simulink model "solution"  (R2017b)
settings: Solver=VariableStepAuto  StartTime=0.0  StopTime=25  FixedStep=0.01  RelTol=1e-3
libraries: simulink x3
settings Model: Creator=ashwin.ramanujam  LastModifiedBy=Vjekoslav

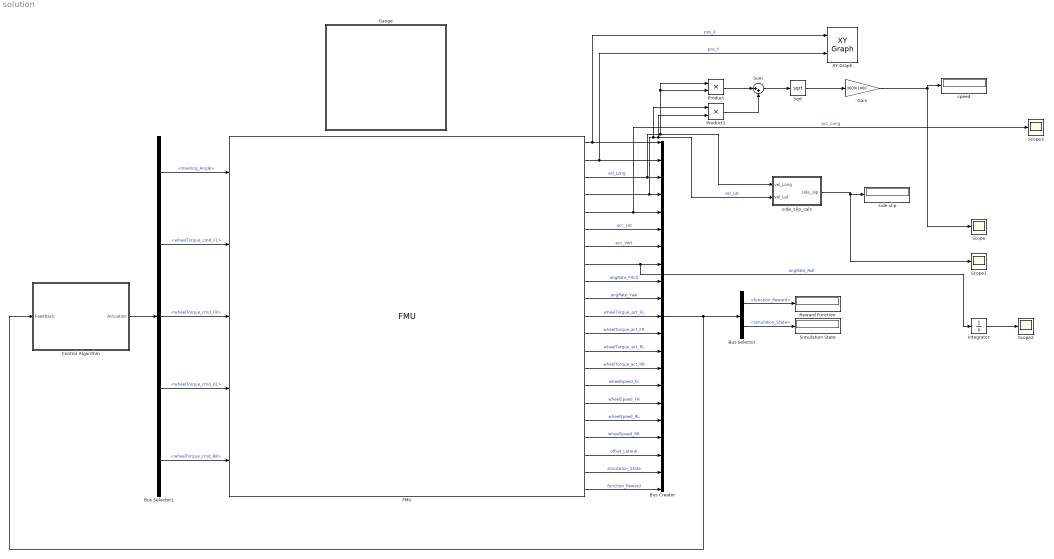
== system solution ==
  Bus Creator : BusCreator  Inputs=21
  Bus Selector : BusSelector  OutputSignals=function_Reward,simulation_State
  Bus Selector1 : BusSelector  OutputSignals=steering_Angle,wheelTorque_cmd_FL,wheelTorque_cmd_FR,wheelTorque_cmd_RL,wheelTorque_cmd_RR
  Control Algorithm : Subsystem
  FMU : FMU  FMUName=MED2018_VehicleModel.fmu  FMUDebugLogging=on  FMUMode=CoSimulation  FMUSampleTime=-1  mask(MED2018.VehicleModel [Co-Simulation, v2.0]){}
      mask Display:
      | if (exist([Simulink.fileGenControl('get','CacheFolder') '\slprj\_fmu\4898b8570ed7ce0a5f76050f8aadaa4c\MED2018_VehicleModel\model.png'],'file'))
      |     image([Simulink.fileGenControl('get','CacheFolder') '\slprj\_fmu\4898b8570ed7ce0a5f76050f8aadaa4c\MED2018_VehicleModel\model.png']);
      |     text(0.03, 0.97, 'MED2018.VehicleModel', 'horizontalAlignment', 'left', 'verticalAlignment', 'top');
      | else
      |     disp('MED2018.VehicleModel');
      | end
      | port_label('output',1,'pos_X');
      | port_label('output',2,'pos_Y');
      | port_label('output',3,'vel_Long');
      | port_label('output',4,'vel_Lat');
      | port_label('output',5,'acc_Long');
      | port_label('output',6,'acc_Lat');
      | port_label('output',7,'acc_Vert');
      | port_label('output',8,'angRate_Roll');
      | port_label('output',9,'angRate_Pitch');
      | port_label('output',10,'angRate_Yaw');
      | port_label('output',11,'wheellTorque_act_FL');
      | port_label('output',12,'wheelTorque_act_FR');
      | port_label('output',13,'wheelTorque_act_RL');
      | port_label('output',14,'wheelTorque_act_RR');
      | port_label('output',15,'wheelSpeed_FL');
      | port_label('output',16,'wheelSpeed_FR');
      | port_label('output',17,'wheelSpeed_RL');
      | port_label('output',18,'wheelSpeed_RR');
      | port_label('output',19,'offset_Lateral');
      | port_label('output',20,'simulation_State');
      | port_label('output',21,'function_Reward');
      | port_label('input',1,'steering_Angle');
      | port_label('input',2,'wheelTorque_cmd_FL');
      | port_label('input',3,'wheelTorque_cmd_FR');
      | port_label('input',4,'wheelTorque_cmd_RL');
      | port_label('input',5,'wheelTorque_cmd_RR');
  Gain : Gain  Gain=3600/1000
  Gauge : Subsystem  DialogController=hmiCreateDDGDialog  IsWebBlock=on  mask(MWDashboardBlock){webBlockId=95ecb222-2df1-432b-9766-14efc8d26a24, webBlockType=circulargauge, ShowInLibBrowser=on, ShowInitialText=on, HMISrcModelName=solution}
      mask prompts: webBlockId "WebBlock Id"; webBlockType "WebBlock Type"; HMISrcModelName "Source Model"
      mask help: SimulinkHMI:dialogs:CircularGaugeDialogDesc
      mask Help: helpview([docroot '/mapfiles/simulink.map'], 'hmi_gauge')
      mask Display:
      | if strcmp(get_param(bdroot(gcb),'BlockDiagramType'), 'library')
      |     image([(matlabroot) '/toolbox/simulink/hmi/icons/CircularGauge.png']);
      | end
  Integrator : Integrator
  Product : Product
  Product1 : Product
  Reward Function : Display
  Scope{,1..3} (4 alike) : Scope
  Simulation State : Display
  Sqrt : Sqrt  SaturateOnIntegerOverflow=on
  Sum : Sum  Inputs=|++
  XY Graph : simulink/Sinks/XY Graph  xmin=-100  xmax=200  ymin=-100  ymax=200  st=-1
  "side slip " : Display
  side_slip_calc : Subsystem
  "speed " : Display
  wires:
  Control Algorithm/1(Actuation) -> Bus Selector1/1
  Bus Selector1/1 -> FMU/1  "<steering_Angle>"
  Bus Selector1/2 -> FMU/2  "<wheelTorque_cmd_FL>"
  Bus Selector1/3 -> FMU/3  "<wheelTorque_cmd_FR>"
  Bus Selector1/4 -> FMU/4  "<wheelTorque_cmd_RL>"
  Bus Selector1/5 -> FMU/5  "<wheelTorque_cmd_RR>"
  FMU/1 -> XY Graph/1, Bus Creator/1  "pos_X"
  FMU/2 -> XY Graph/2, Bus Creator/2  "pos_Y"
  FMU/3 -> side_slip_calc/1(vel_Long), Product/2, Product/1, Bus Creator/3  "vel_Long"
  FMU/4 -> Product1/1, side_slip_calc/2(vel_Lat), Product1/2, Bus Creator/4  "vel_Lat"
  FMU/5 -> Scope3/1, Bus Creator/5  "acc_Long"
  FMU/6 -> Bus Creator/6  "acc_Lat"
  FMU/7 -> Bus Creator/7  "acc_Vert"
  FMU/8 -> Integrator/1, Bus Creator/8  "angRate_Roll"
  FMU/9 -> Bus Creator/9  "angRate_Pitch"
  FMU/10 -> Bus Creator/10  "angRate_Yaw"
  FMU/11 -> Bus Creator/11  "wheelTorque_act_FL"
  FMU/12 -> Bus Creator/12  "wheelTorque_act_FR"
  FMU/13 -> Bus Creator/13  "wheelTorque_act_RL"
  FMU/14 -> Bus Creator/14  "wheelTorque_act_RR"
  FMU/15 -> Bus Creator/15  "wheelSpeed_FL"
  FMU/16 -> Bus Creator/16  "wheelSpeed_FR"
  FMU/17 -> Bus Creator/17  "wheelSpeed_RL"
  FMU/18 -> Bus Creator/18  "wheelSpeed_RR"
  FMU/19 -> Bus Creator/19  "offset_Lateral"
  FMU/20 -> Bus Creator/20  "simulation_State"
  FMU/21 -> Bus Creator/21  "function_Reward"
  Bus Creator/1 -> Bus Selector/1, Control Algorithm/1(Feedback)
  Bus Selector/1 -> Reward Function/1  "<function_Reward>"
  Bus Selector/2 -> Simulation State/1  "<simulation_State>"
  Product1/1 -> Sum/2
  Product/1 -> Sum/1
  Sum/1 -> Sqrt/1
  Sqrt/1 -> Gain/1
  Gain/1 -> "speed "/1, Scope/1
  Integrator/1 -> Scope2/1
  side_slip_calc/1(side_slip) -> Scope1/1, "side slip "/1

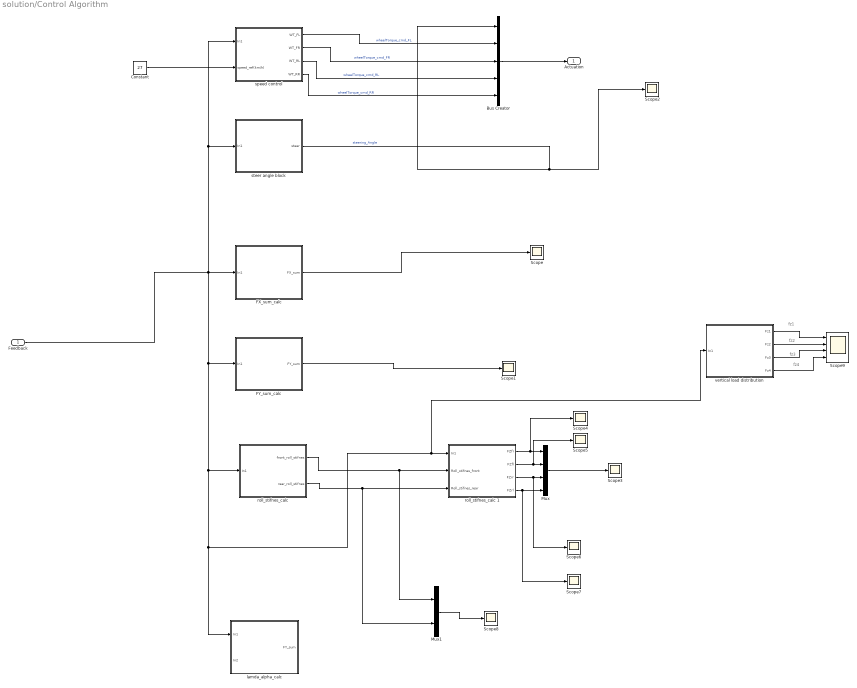
== system solution/Control Algorithm ==
  note: fz3
  note: fz4
  note: fz1
  note: fz2
  Feedback : Inport
  Bus Creator : BusCreator  Inputs=5
  Constant : Constant  Value=27
  FX_sum_calc : Subsystem
  FY_sum_calc : Subsystem
  Mux : Mux
  Mux1 : Mux  Inputs=2
  Scope{,1..8} (9 alike) : Scope
  Scope9 : Scope  NumInputPorts=4
  lamda_alpha_calc : Subsystem
  "roll_stifnes_calc " : Subsystem
  roll_stifnes_calc 1 : Subsystem
  speed control : Subsystem
  "steer angle block " : Subsystem
  vertical load distribution : Subsystem
  Actuation : Outport
  wires:
  speed control/4(WT_RR) -> Bus Creator/5  "wheelTorque_cmd_RR"
  speed control/1("WT_FL ") -> Bus Creator/2  "wheelTorque_cmd_FL"
  speed control/3(WT_RL) -> Bus Creator/4  "wheelTorque_cmd_RL"
  "steer angle block "/1("steer ") -> Scope2/1, Bus Creator/1  "steering_Angle"
  speed control/2(WT_FR) -> Bus Creator/3  "wheelTorque_cmd_FR"
  Bus Creator/1 -> Actuation/1
  FX_sum_calc/1(FX_sum) -> Scope/1
  FY_sum_calc/1(FY_sum) -> Scope1/1
  "roll_stifnes_calc "/1(front_roll_stifnes) -> Mux1/1, roll_stifnes_calc 1/2(Roll_stifnes_front)
  "roll_stifnes_calc "/2(rear_roll_stifnes) -> Mux1/2, roll_stifnes_calc 1/3("Roll_stifnes_rear ")
  Constant/1 -> speed control/2("speed_ref(km/h) ")
  roll_stifnes_calc 1/1(FZfr) -> Scope4/1, Mux/1
  roll_stifnes_calc 1/2(FZfl) -> Scope5/1, Mux/2
  roll_stifnes_calc 1/3(FZrr) -> Scope6/1, Mux/3
  roll_stifnes_calc 1/4(FZrl) -> Scope7/1, Mux/4
  Mux/1 -> Scope3/1
  Mux1/1 -> Scope8/1
  vertical load distribution/3(Fz3) -> Scope9/3
  vertical load distribution/4(Fz4) -> Scope9/4
  vertical load distribution/2(Fz2) -> Scope9/2
  vertical load distribution/1(Fz1) -> Scope9/1
  Feedback/1 -> speed control/1(In1), "steer angle block "/1(In1), FY_sum_calc/1(In1), "roll_stifnes_calc "/1(In1), vertical load distribution/1(In1), roll_stifnes_calc 1/1(In1), lamda_alpha_calc/1(In1), FX_sum_calc/1(In1)

== system solution/Gauge ==

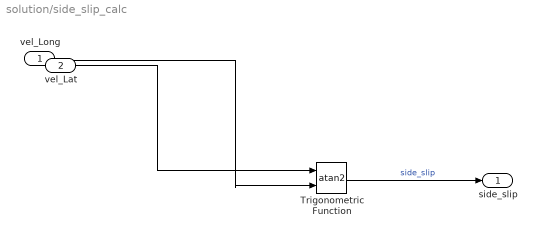
== system solution/side_slip_calc ==
  vel_Long : Inport
  vel_Lat : Inport  Port=2
  Trigonometric Function : Trigonometry  Operator=atan2
  side_slip : Outport
  wires:
  Trigonometric Function/1 -> side_slip/1  "side_slip"
  vel_Lat/1 -> Trigonometric Function/1
  vel_Long/1 -> Trigonometric Function/2

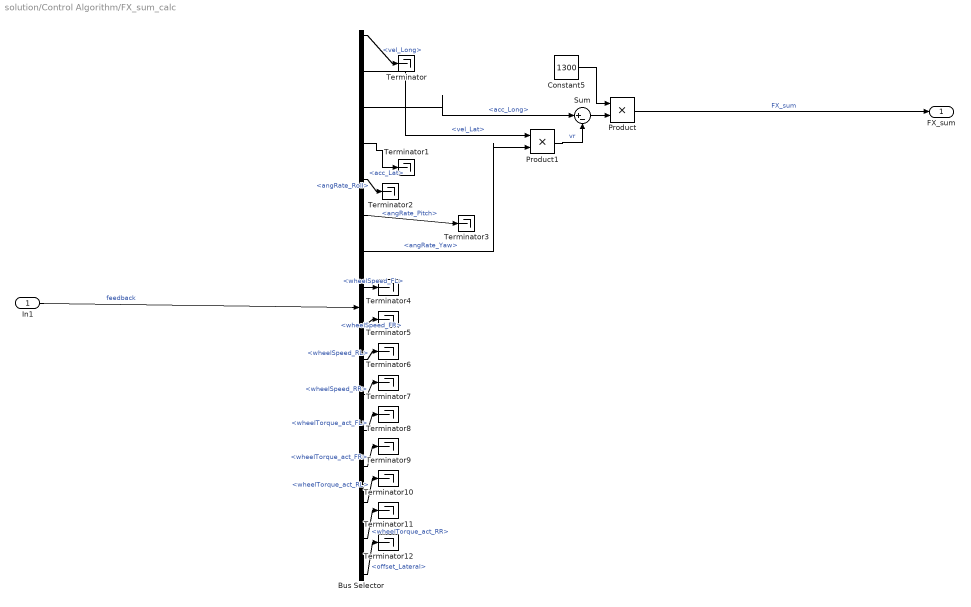
== system solution/Control Algorithm/FX_sum_calc ==
  In1 : Inport
  Bus Selector : BusSelector  OutputSignals=vel_Long,vel_Lat,acc_Long,acc_Lat,angRate_Roll,angRate_Pitch,angRate_Yaw,wheelSpeed_FL,wheelSpeed_FR,wheelSpeed_RL,wheelSpeed_RR,wheelTorque_act_FL,wheelTorque_act_FR,wheelTorque_act_RL,wheelTorque_act_RR,offset_Lateral
  Constant5 : Constant  Value=1300
  Product : Product
  Product1 : Product
  Sum : Sum  Inputs=|+-
  Terminator{,1..12} (13 alike) : Terminator
  FX_sum : Outport
  wires:
  Constant5/1 -> Product/1
  Product1/1 -> Sum/2  "vr"
  Product/1 -> FX_sum/1  "FX_sum"
  Bus Selector/7 -> Product1/2  "<angRate_Yaw>"
  Bus Selector/3 -> Sum/1  "<acc_Long>"
  Bus Selector/6 -> Terminator3/1  "<angRate_Pitch>"
  Bus Selector/10 -> Terminator6/1  "<wheelSpeed_RL>"
  Bus Selector/8 -> Terminator4/1  "<wheelSpeed_FL>"
  Bus Selector/9 -> Terminator5/1  "<wheelSpeed_FR>"
  Bus Selector/15 -> Terminator11/1  "<wheelTorque_act_RR>"
  Bus Selector/16 -> Terminator12/1  "<offset_Lateral>"
  Bus Selector/12 -> Terminator8/1  "<wheelTorque_act_FL>"
  Bus Selector/11 -> Terminator7/1  "<wheelSpeed_RR>"
  Bus Selector/14 -> Terminator10/1  "<wheelTorque_act_RL>"
  Bus Selector/1 -> Terminator/1  "<vel_Long>"
  Bus Selector/5 -> Terminator2/1  "<angRate_Roll>"
  Bus Selector/13 -> Terminator9/1  "<wheelTorque_act_FR>"
  Bus Selector/4 -> Terminator1/1  "<acc_Lat>"
  Bus Selector/2 -> Product1/1  "<vel_Lat>"
  In1/1 -> Bus Selector/1  "feedback"
  Sum/1 -> Product/2

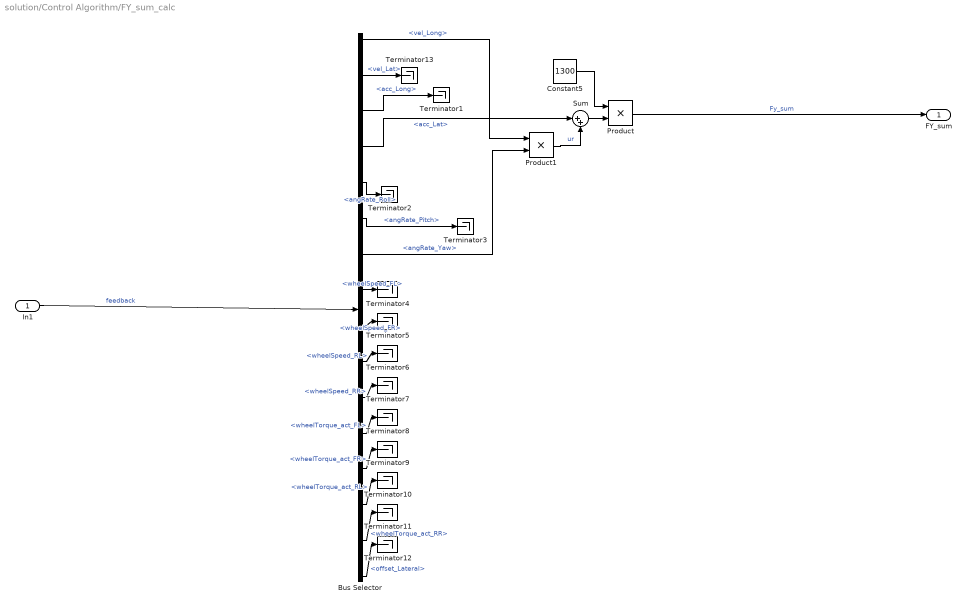
== system solution/Control Algorithm/FY_sum_calc ==
  In1 : Inport
  Bus Selector : BusSelector  OutputSignals=vel_Long,vel_Lat,acc_Long,acc_Lat,angRate_Roll,angRate_Pitch,angRate_Yaw,wheelSpeed_FL,wheelSpeed_FR,wheelSpeed_RL,wheelSpeed_RR,wheelTorque_act_FL,wheelTorque_act_FR,wheelTorque_act_RL,wheelTorque_act_RR,offset_Lateral
  Constant5 : Constant  Value=1300
  Product : Product
  Product1 : Product
  Sum : Sum  Inputs=|++
  Terminator{1..13} (13 alike) : Terminator
  FY_sum : Outport
  wires:
  Sum/1 -> Product/2
  In1/1 -> Bus Selector/1  "feedback"
  Bus Selector/4 -> Sum/1  "<acc_Lat>"
  Bus Selector/13 -> Terminator9/1  "<wheelTorque_act_FR>"
  Bus Selector/5 -> Terminator2/1  "<angRate_Roll>"
  Bus Selector/1 -> Product1/1  "<vel_Long>"
  Bus Selector/14 -> Terminator10/1  "<wheelTorque_act_RL>"
  Bus Selector/11 -> Terminator7/1  "<wheelSpeed_RR>"
  Bus Selector/12 -> Terminator8/1  "<wheelTorque_act_FL>"
  Bus Selector/16 -> Terminator12/1  "<offset_Lateral>"
  Bus Selector/15 -> Terminator11/1  "<wheelTorque_act_RR>"
  Bus Selector/9 -> Terminator5/1  "<wheelSpeed_FR>"
  Bus Selector/8 -> Terminator4/1  "<wheelSpeed_FL>"
  Bus Selector/10 -> Terminator6/1  "<wheelSpeed_RL>"
  Bus Selector/6 -> Terminator3/1  "<angRate_Pitch>"
  Bus Selector/7 -> Product1/2  "<angRate_Yaw>"
  Product/1 -> FY_sum/1  "Fy_sum"
  Product1/1 -> Sum/2  "ur"
  Constant5/1 -> Product/1
  Bus Selector/3 -> Terminator1/1  "<acc_Long>"
  Bus Selector/2 -> Terminator13/1  "<vel_Lat>"

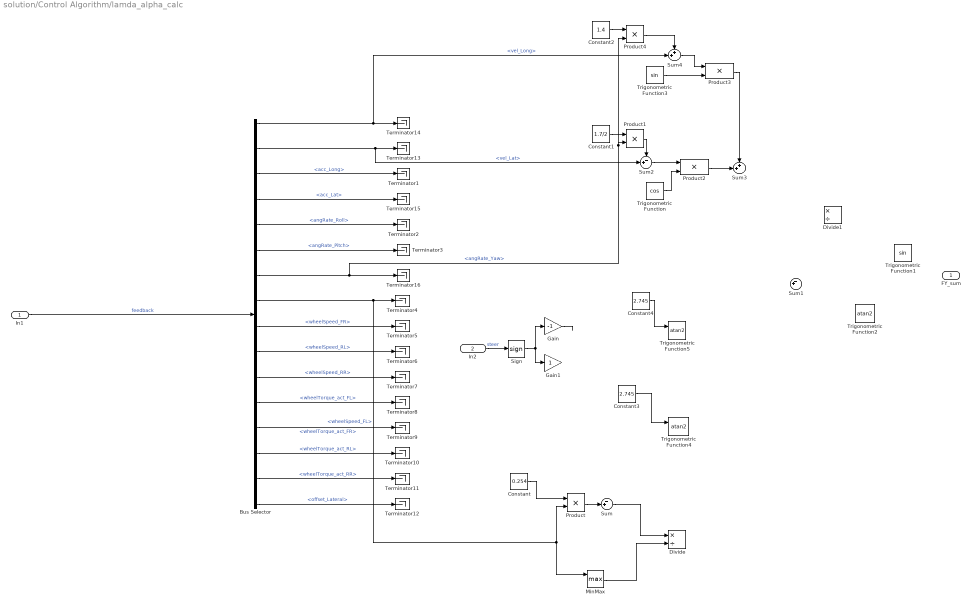
== system solution/Control Algorithm/lamda_alpha_calc ==
  In1 : Inport
  In2 : Inport  Port=2
  Bus Selector : BusSelector  OutputSignals=vel_Long,vel_Lat,acc_Long,acc_Lat,angRate_Roll,angRate_Pitch,angRate_Yaw,wheelSpeed_FL,wheelSpeed_FR,wheelSpeed_RL,wheelSpeed_RR,wheelTorque_act_FL,wheelTorque_act_FR,wheelTorque_act_RL,wheelTorque_act_RR,offset_Lateral
  Constant : Constant  Value=0.254
  Constant1 : Constant  Value=1.7/2
  Constant2 : Constant  Value=1.4
  Constant3 : Constant  Value=2.745
  Constant4 : Constant  Value=2.745
  Divide : Product  Inputs=*/
  Divide1 : Product  Inputs=*/
  Gain : Gain  Gain=-1
  Gain1 : Gain
  MinMax : MinMax  Function=max  Inputs=2
  Product{,1..4} (5 alike) : Product
  Sign : Signum
  Sum : Sum  Inputs=-+|
  Sum1 : Sum  Inputs=-+|
  Sum2 : Sum  Inputs=-+|
  Sum3 : Sum  Inputs=++|
  Sum4 : Sum  Inputs=++|
  Terminator{1..16} (16 alike) : Terminator
  Trigonometric Function : Trigonometry  Operator=cos
  Trigonometric Function1 : Trigonometry
  Trigonometric Function2 : Trigonometry  Operator=atan2
  Trigonometric Function3 : Trigonometry
  Trigonometric Function4 : Trigonometry  Operator=atan2
  Trigonometric Function5 : Trigonometry  Operator=atan2
  FY_sum : Outport
  wires:
  Bus Selector/2 -> Sum2/2, Terminator13/1  "<vel_Lat>"
  Bus Selector/3 -> Terminator1/1  "<acc_Long>"
  Bus Selector/6 -> Terminator3/1  "<angRate_Pitch>"
  Bus Selector/10 -> Terminator6/1  "<wheelSpeed_RL>"
  Bus Selector/8 -> MinMax/1, Product/2, Terminator4/1  "<wheelSpeed_FL>"
  Bus Selector/9 -> Terminator5/1  "<wheelSpeed_FR>"
  Bus Selector/15 -> Terminator11/1  "<wheelTorque_act_RR>"
  Bus Selector/16 -> Terminator12/1  "<offset_Lateral>"
  Bus Selector/12 -> Terminator8/1  "<wheelTorque_act_FL>"
  Bus Selector/11 -> Terminator7/1  "<wheelSpeed_RR>"
  Bus Selector/14 -> Terminator10/1  "<wheelTorque_act_RL>"
  Bus Selector/5 -> Terminator2/1  "<angRate_Roll>"
  Bus Selector/13 -> Terminator9/1  "<wheelTorque_act_FR>"
  In1/1 -> Bus Selector/1  "feedback"
  Bus Selector/1 -> Sum4/2, Terminator14/1  "<vel_Long>"
  Bus Selector/4 -> Terminator15/1  "<acc_Lat>"
  Bus Selector/7 -> Product4/2, Product1/2, Terminator16/1  "<angRate_Yaw>"
  MinMax/1 -> Divide/2
  Constant/1 -> Product/1
  Product/1 -> Sum/2
  Sum/1 -> Divide/1
  ? -> MinMax/2, Sum/1
  Constant1/1 -> Product1/1
  Product1/1 -> Sum2/1
  Sum2/1 -> Product2/1
  Trigonometric Function/1 -> Product2/2
  Product2/1 -> Sum3/2
  Trigonometric Function3/1 -> Product3/2
  Sum4/1 -> Product3/1
  Product3/1 -> Sum3/1
  Constant2/1 -> Product4/1
  Product4/1 -> Sum4/1
  ? -> Trigonometric Function/1
  ? -> Trigonometric Function3/1
  Constant3/1 -> Trigonometric Function4/1
  In2/1 -> Sign/1  "steer"
  Sign/1 -> Gain1/1, Gain/1
  Gain/1 -> ?
  Constant4/1 -> Trigonometric Function5/1

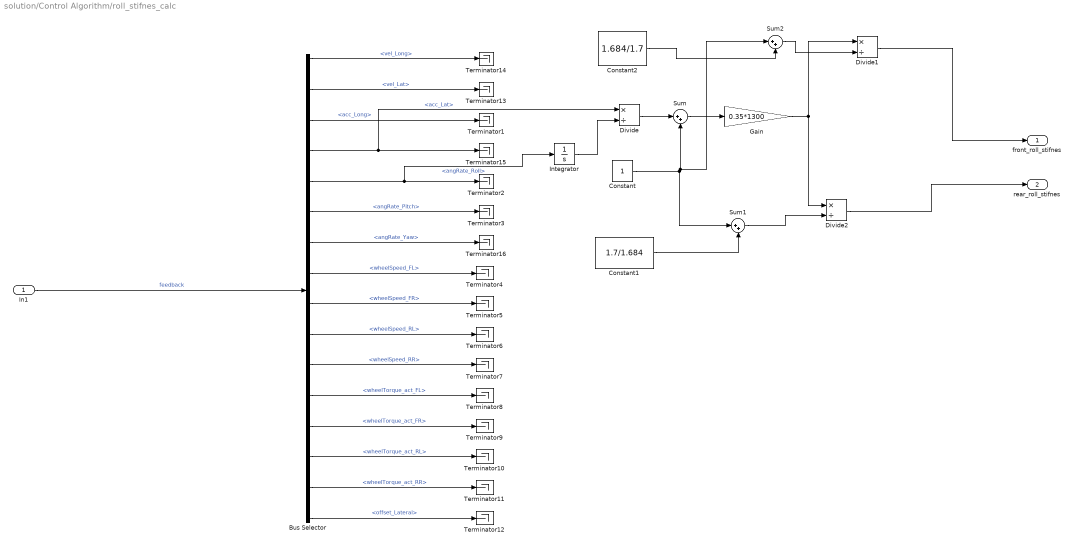
== system solution/Control Algorithm/roll_stifnes_calc  ==
  In1 : Inport
  Bus Selector : BusSelector  OutputSignals=vel_Long,vel_Lat,acc_Long,acc_Lat,angRate_Roll,angRate_Pitch,angRate_Yaw,wheelSpeed_FL,wheelSpeed_FR,wheelSpeed_RL,wheelSpeed_RR,wheelTorque_act_FL,wheelTorque_act_FR,wheelTorque_act_RL,wheelTorque_act_RR,offset_Lateral
  Constant : Constant
  Constant1 : Constant  Value=1.7/1.684
  Constant2 : Constant  Value=1.684/1.7
  Divide : Product  Inputs=*/
  Divide1 : Product  Inputs=*/
  Divide2 : Product  Inputs=*/
  Gain : Gain  Gain=0.35*1300
  Integrator : Integrator
  Sum : Sum  Inputs=|++
  Sum1 : Sum  Inputs=|++
  Sum2 : Sum  Inputs=|++
  Terminator{1..16} (16 alike) : Terminator
  front_roll_stifnes : Outport
  rear_roll_stifnes : Outport  Port=2
  wires:
  Bus Selector/7 -> Terminator16/1  "<angRate_Yaw>"
  Bus Selector/4 -> Divide/1, Terminator15/1  "<acc_Lat>"
  Bus Selector/1 -> Terminator14/1  "<vel_Long>"
  In1/1 -> Bus Selector/1  "feedback"
  Bus Selector/13 -> Terminator9/1  "<wheelTorque_act_FR>"
  Bus Selector/5 -> Integrator/1, Terminator2/1  "<angRate_Roll>"
  Bus Selector/14 -> Terminator10/1  "<wheelTorque_act_RL>"
  Bus Selector/11 -> Terminator7/1  "<wheelSpeed_RR>"
  Bus Selector/12 -> Terminator8/1  "<wheelTorque_act_FL>"
  Bus Selector/16 -> Terminator12/1  "<offset_Lateral>"
  Bus Selector/15 -> Terminator11/1  "<wheelTorque_act_RR>"
  Bus Selector/9 -> Terminator5/1  "<wheelSpeed_FR>"
  Bus Selector/8 -> Terminator4/1  "<wheelSpeed_FL>"
  Bus Selector/10 -> Terminator6/1  "<wheelSpeed_RL>"
  Bus Selector/6 -> Terminator3/1  "<angRate_Pitch>"
  Bus Selector/3 -> Terminator1/1  "<acc_Long>"
  Bus Selector/2 -> Terminator13/1  "<vel_Lat>"
  Integrator/1 -> Divide/2
  Constant/1 -> Sum1/1, Sum2/1, Sum/2
  Divide/1 -> Sum/1
  Sum/1 -> Gain/1
  Gain/1 -> Divide2/1, Divide1/1
  Sum2/1 -> Divide1/2
  Sum1/1 -> Divide2/2
  Constant1/1 -> Sum1/2
  Constant2/1 -> Sum2/2
  Divide1/1 -> front_roll_stifnes/1
  Divide2/1 -> rear_roll_stifnes/1

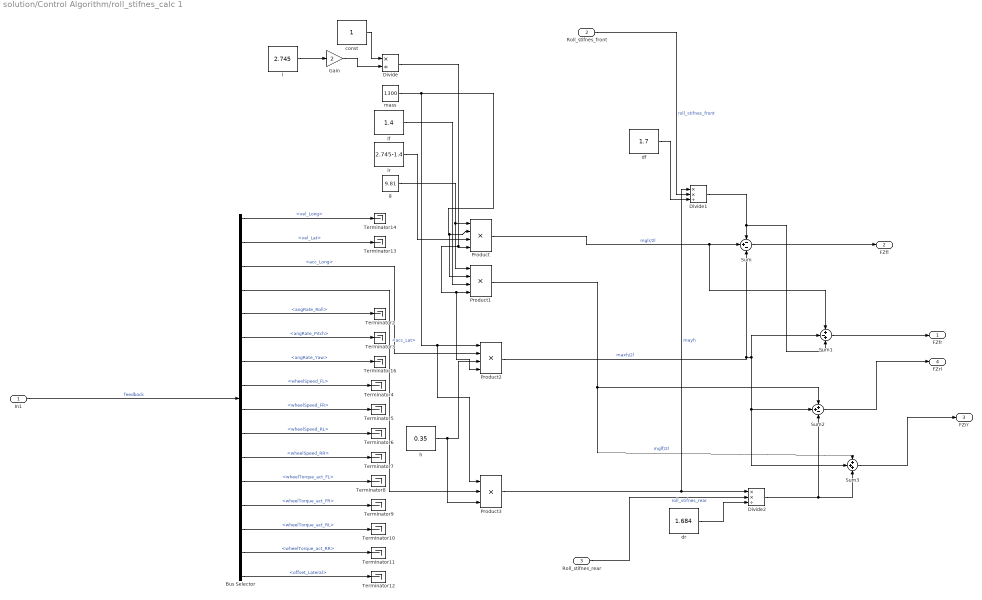
== system solution/Control Algorithm/roll_stifnes_calc 1 ==
  In1 : Inport
  Roll_stifnes_front : Inport  Port=2
  "Roll_stifnes_rear " : Inport  Port=3
  Bus Selector : BusSelector  OutputSignals=vel_Long,vel_Lat,acc_Long,acc_Lat,angRate_Roll,angRate_Pitch,angRate_Yaw,wheelSpeed_FL,wheelSpeed_FR,wheelSpeed_RL,wheelSpeed_RR,wheelTorque_act_FL,wheelTorque_act_FR,wheelTorque_act_RL,wheelTorque_act_RR,offset_Lateral
  Divide : Product  Inputs=*/
  Divide1 : Product  Inputs=**/
  Divide2 : Product  Inputs=**/
  Gain : Gain  Gain=2
  Product : Product  Inputs=4
  Product1 : Product  Inputs=4
  Product2 : Product  Inputs=4
  Product3 : Product  Inputs=3
  Sum : Sum  Inputs=-+-
  Sum1 : Sum  Inputs=+-+
  Sum2 : Sum  Inputs=++-
  Sum3 : Sum  Inputs=+++
  Terminator{2..14,16} (14 alike) : Terminator
  const : Constant
  df : Constant  Value=1.7
  dr : Constant  Value=1.684
  g : Constant  Value=9.81
  h : Constant  Value=0.35
  "l " : Constant  Value=2.745
  "lf " : Constant  Value=1.4
  lr : Constant  Value=2.745-1.4
  mass : Constant  Value=1300
  FZfr : Outport
  FZfl : Outport  Port=2
  FZrr : Outport  Port=3
  FZrl : Outport  Port=4
  wires:
  Bus Selector/2 -> Terminator13/1  "<vel_Lat>"
  Bus Selector/3 -> Product2/2  "<acc_Long>"
  Bus Selector/6 -> Terminator3/1  "<angRate_Pitch>"
  Bus Selector/10 -> Terminator6/1  "<wheelSpeed_RL>"
  Bus Selector/8 -> Terminator4/1  "<wheelSpeed_FL>"
  Bus Selector/9 -> Terminator5/1  "<wheelSpeed_FR>"
  Bus Selector/15 -> Terminator11/1  "<wheelTorque_act_RR>"
  Bus Selector/16 -> Terminator12/1  "<offset_Lateral>"
  Bus Selector/12 -> Terminator8/1  "<wheelTorque_act_FL>"
  Bus Selector/11 -> Terminator7/1  "<wheelSpeed_RR>"
  Bus Selector/14 -> Terminator10/1  "<wheelTorque_act_RL>"
  Bus Selector/5 -> Terminator2/1  "<angRate_Roll>"
  Bus Selector/13 -> Terminator9/1  "<wheelTorque_act_FR>"
  In1/1 -> Bus Selector/1  "feedback"
  Bus Selector/1 -> Terminator14/1  "<vel_Long>"
  Bus Selector/4 -> Product3/2  "<acc_Lat>"
  Bus Selector/7 -> Terminator16/1  "<angRate_Yaw>"
  Roll_stifnes_front/1 -> Divide1/2  "roll_stifnes_front"
  "Roll_stifnes_rear "/1 -> Divide2/2  "roll_stifnes_rear"
  g/1 -> Product1/1, Product/1
  mass/1 -> Product3/1, Product2/1, Product1/2, Product/2
  lr/1 -> Product/3
  "lf "/1 -> Product1/3
  Product1/1 -> Sum3/1, Sum2/1  "mglf/2l"
  "l "/1 -> Gain/1
  const/1 -> Divide/1
  Gain/1 -> Divide/2
  Divide/1 -> Product2/4, Product1/4, Product/4
  h/1 -> Product3/3, Product2/3
  Product2/1 -> Sum3/2, Sum2/2, Sum1/2, Sum/3  "maxh/2l"
  Product3/1 -> Divide2/1, Divide1/1  "mayh"
  Sum/1 -> FZfl/1
  Product/1 -> Sum1/1, Sum/2  "mglr/2l"
  df/1 -> Divide1/3
  Divide1/1 -> Sum1/3, Sum/1
  Sum1/1 -> FZfr/1
  Sum2/1 -> FZrl/1
  Divide2/1 -> Sum3/3, Sum2/3
  dr/1 -> Divide2/3
  Sum3/1 -> FZrr/1

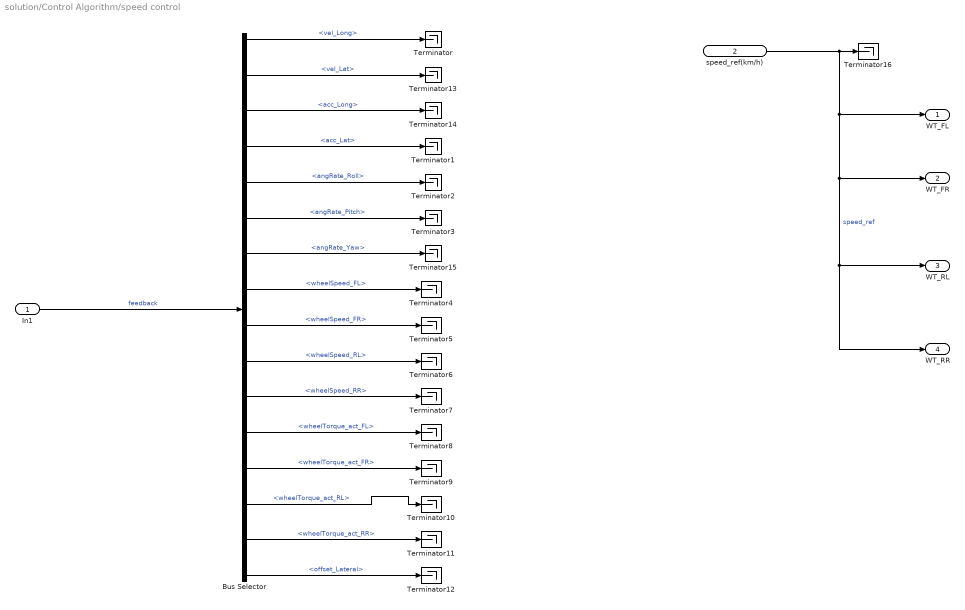
== system solution/Control Algorithm/speed control ==
  In1 : Inport
  "speed_ref(km/h) " : Inport  Port=2
  Bus Selector : BusSelector  OutputSignals=vel_Long,vel_Lat,acc_Long,acc_Lat,angRate_Roll,angRate_Pitch,angRate_Yaw,wheelSpeed_FL,wheelSpeed_FR,wheelSpeed_RL,wheelSpeed_RR,wheelTorque_act_FL,wheelTorque_act_FR,wheelTorque_act_RL,wheelTorque_act_RR,offset_Lateral
  Terminator{,1..16} (17 alike) : Terminator
  "WT_FL " : Outport
  WT_FR : Outport  Port=2
  WT_RL : Outport  Port=3
  WT_RR : Outport  Port=4
  wires:
  Bus Selector/7 -> Terminator15/1  "<angRate_Yaw>"
  Bus Selector/2 -> Terminator13/1  "<vel_Lat>"
  Bus Selector/3 -> Terminator14/1  "<acc_Long>"
  Bus Selector/6 -> Terminator3/1  "<angRate_Pitch>"
  Bus Selector/10 -> Terminator6/1  "<wheelSpeed_RL>"
  Bus Selector/8 -> Terminator4/1  "<wheelSpeed_FL>"
  Bus Selector/9 -> Terminator5/1  "<wheelSpeed_FR>"
  Bus Selector/15 -> Terminator11/1  "<wheelTorque_act_RR>"
  Bus Selector/16 -> Terminator12/1  "<offset_Lateral>"
  Bus Selector/12 -> Terminator8/1  "<wheelTorque_act_FL>"
  Bus Selector/11 -> Terminator7/1  "<wheelSpeed_RR>"
  Bus Selector/14 -> Terminator10/1  "<wheelTorque_act_RL>"
  Bus Selector/1 -> Terminator/1  "<vel_Long>"
  Bus Selector/5 -> Terminator2/1  "<angRate_Roll>"
  Bus Selector/13 -> Terminator9/1  "<wheelTorque_act_FR>"
  Bus Selector/4 -> Terminator1/1  "<acc_Lat>"
  In1/1 -> Bus Selector/1  "feedback"
  "speed_ref(km/h) "/1 -> WT_RR/1, WT_RL/1, WT_FR/1, "WT_FL "/1, Terminator16/1  "speed_ref"

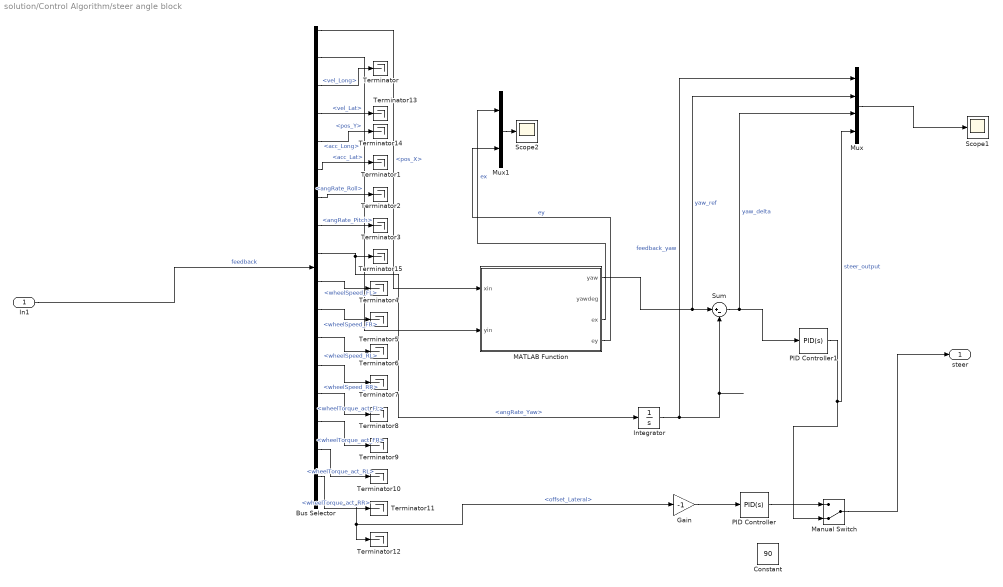
== system solution/Control Algorithm/steer angle block  ==
  In1 : Inport
  Bus Selector : BusSelector  OutputSignals=pos_X,pos_Y,vel_Long,vel_Lat,acc_Long,acc_Lat,angRate_Roll,angRate_Pitch,angRate_Yaw,wheelSpeed_FL,wheelSpeed_FR,wheelSpeed_RL,wheelSpeed_RR,wheelTorque_act_FL,wheelTorque_act_FR,wheelTorque_act_RL,wheelTorque_act_RR,offset_Lateral
  Constant : Constant  Value=90
  Gain : Gain  Gain=-1
  Integrator : Integrator
  MATLAB Function : MATLAB Function  TreatAsAtomicUnit=on
  Manual Switch : ManualSwitch  CurrentSetting=0
  Mux : Mux
  Mux1 : Mux  Inputs=2
  PID Controller : simulink/Continuous/PID Controller  Controller=PID  TimeDomain=Continuous-time  SampleTime=-1  IntegratorMethod=Forward Euler  FilterMethod=Forward Euler  Form=Parallel  UseFilter=on  ControllerParametersSource=internal  P=1  I=0  D=1  N=100  InitialConditionSource=internal  InitialConditionForIntegrator=0  InitialConditionForFilter=0  ExternalReset=none  LimitOutput=off  UpperSaturationLimit=inf  LowerSaturationLimit=-inf  LinearizeAsGain=on  AntiWindupMode=none  Kb=1  TrackingMode=off  Kt=1  PParamMin=[]  PParamMax=[]  IParamMin=[]  IParamMax=[]  DParamMin=[]  DParamMax=[]  NParamMin=[]  NParamMax=[]  KbParamMin=[]  KbParamMax=[]  KtParamMin=[]  KtParamMax=[]  POutMin=[]  POutMax=[]  IOutMin=[]  IOutMax=[]  DOutMin=[]  DOutMax=[]  NOutMin=[]  NOutMax=[]  KbOutMin=[]  KbOutMax=[]  KtOutMin=[]  KtOutMax=[]  IntegratorOutMin=[]  IntegratorOutMax=[]  FilterOutMin=[]  FilterOutMax=[]  SumOutMin=[]  SumOutMax=[]  SumI1OutMin=[]  SumI1OutMax=[]  SumI2OutMin=[]  SumI2OutMax=[]  SumI3OutMin=[]  SumI3OutMax=[]  SumDOutMin=[]  SumDOutMax=[]  SaturationOutMin=[]  SaturationOutMax=[]  IntegratorContinuousStateAttributes=''  IntegratorStateMustResolveToSignalObject=off  IntegratorRTWStateStorageClass=Auto  FilterContinuousStateAttributes=''  FilterStateMustResolveToSignalObject=off  FilterRTWStateStorageClass=Auto  DifferentiatorICPrevScaledInput=0  DifferentiatorOutMin=[]  DifferentiatorOutMax=[]  InitialConditionSetting=State (most efficient)  FilterDiffOutCoefMin=[]  FilterDiffOutCoefMax=[]  SumDenOutMin=[]  SumDenOutMax=[]  SumNumOutMin=[]  SumNumOutMax=[]  ReciprocalOutMin=[]  ReciprocalOutMax=[]  DivideOutMin=[]  DivideOutMax=[]  TunerSelectOption=Transfer Function Based (PID Tuner App)
  PID Controller1 : simulink/Continuous/PID Controller  Controller=PID  TimeDomain=Continuous-time  SampleTime=-1  IntegratorMethod=Forward Euler  FilterMethod=Forward Euler  Form=Parallel  UseFilter=on  ControllerParametersSource=internal  P=10  I=5  D=5  N=0  InitialConditionSource=internal  InitialConditionForIntegrator=0  InitialConditionForFilter=0  ExternalReset=none  LimitOutput=off  UpperSaturationLimit=inf  LowerSaturationLimit=-inf  LinearizeAsGain=on  AntiWindupMode=none  Kb=1  TrackingMode=off  Kt=1  PParamMin=[]  PParamMax=[]  IParamMin=[]  IParamMax=[]  DParamMin=[]  DParamMax=[]  NParamMin=[]  NParamMax=[]  KbParamMin=[]  KbParamMax=[]  KtParamMin=[]  KtParamMax=[]  POutMin=[]  POutMax=[]  IOutMin=[]  IOutMax=[]  DOutMin=[]  DOutMax=[]  NOutMin=[]  NOutMax=[]  KbOutMin=[]  KbOutMax=[]  KtOutMin=[]  KtOutMax=[]  IntegratorOutMin=[]  IntegratorOutMax=[]  FilterOutMin=[]  FilterOutMax=[]  SumOutMin=[]  SumOutMax=[]  SumI1OutMin=[]  SumI1OutMax=[]  SumI2OutMin=[]  SumI2OutMax=[]  SumI3OutMin=[]  SumI3OutMax=[]  SumDOutMin=[]  SumDOutMax=[]  SaturationOutMin=[]  SaturationOutMax=[]  IntegratorContinuousStateAttributes=''  IntegratorStateMustResolveToSignalObject=off  IntegratorRTWStateStorageClass=Auto  FilterContinuousStateAttributes=''  FilterStateMustResolveToSignalObject=off  FilterRTWStateStorageClass=Auto  DifferentiatorICPrevScaledInput=0  DifferentiatorOutMin=[]  DifferentiatorOutMax=[]  InitialConditionSetting=State (most efficient)  FilterDiffOutCoefMin=[]  FilterDiffOutCoefMax=[]  SumDenOutMin=[]  SumDenOutMax=[]  SumNumOutMin=[]  SumNumOutMax=[]  ReciprocalOutMin=[]  ReciprocalOutMax=[]  DivideOutMin=[]  DivideOutMax=[]  TunerSelectOption=Transfer Function Based (PID Tuner App)
  Scope1 : Scope
  Scope2 : Scope
  Sum : Sum  Inputs=|+-
  Terminator{,1..15} (16 alike) : Terminator
  "steer " : Outport
  wires:
  In1/1 -> Bus Selector/1  "feedback"
  Bus Selector/6 -> Terminator1/1  "<acc_Lat>"
  Bus Selector/15 -> Terminator9/1  "<wheelTorque_act_FR>"
  Bus Selector/7 -> Terminator2/1  "<angRate_Roll>"
  Bus Selector/3 -> Terminator/1  "<vel_Long>"
  Bus Selector/16 -> Terminator10/1  "<wheelTorque_act_RL>"
  Bus Selector/13 -> Terminator7/1  "<wheelSpeed_RR>"
  Bus Selector/14 -> Terminator8/1  "<wheelTorque_act_FL>"
  Bus Selector/18 -> Terminator12/1, Gain/1  "<offset_Lateral>"
  Bus Selector/17 -> Terminator11/1  "<wheelTorque_act_RR>"
  Bus Selector/11 -> Terminator5/1  "<wheelSpeed_FR>"
  Bus Selector/10 -> Terminator4/1  "<wheelSpeed_FL>"
  Bus Selector/12 -> Terminator6/1  "<wheelSpeed_RL>"
  Bus Selector/8 -> Terminator3/1  "<angRate_Pitch>"
  Bus Selector/5 -> Terminator14/1  "<acc_Long>"
  Bus Selector/9 -> Integrator/1, Terminator15/1  "<angRate_Yaw>"
  Gain/1 -> PID Controller/1
  PID Controller/1 -> Manual Switch/1
  Manual Switch/1 -> "steer "/1
  Integrator/1 -> Mux/1, Sum/2  "feedback_yaw"
  MATLAB Function/1(yaw) -> Mux/2, Sum/1  "yaw_ref"
  Sum/1 -> Mux/3, PID Controller1/1  "yaw_delta"
  Bus Selector/1 -> MATLAB Function/1(xin)  "<pos_X>"
  Bus Selector/2 -> MATLAB Function/2(yin)  "<pos_Y>"
  Bus Selector/4 -> Terminator13/1  "<vel_Lat>"
  PID Controller1/1 -> Mux/4, Manual Switch/2  "steer_output"
  Mux/1 -> Scope1/1
  MATLAB Function/3(ex) -> Mux1/1  "ex"
  MATLAB Function/4(ey) -> Mux1/2  "ey"
  Mux1/1 -> Scope2/1

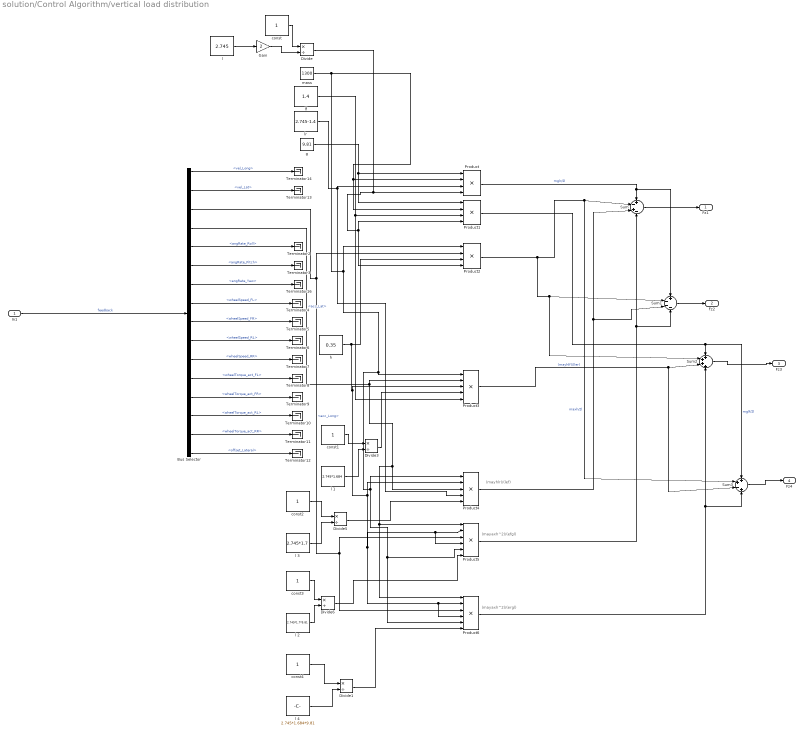
== system solution/Control Algorithm/vertical load distribution ==
  note: (mayaxh^2)/(ergl)
  note: (mayaxh^2)/(efgl)
  note: (mayhlr)/(lef)
  In1 : Inport
  Bus Selector : BusSelector  OutputSignals=vel_Long,vel_Lat,acc_Long,acc_Lat,angRate_Roll,angRate_Pitch,angRate_Yaw,wheelSpeed_FL,wheelSpeed_FR,wheelSpeed_RL,wheelSpeed_RR,wheelTorque_act_FL,wheelTorque_act_FR,wheelTorque_act_RL,wheelTorque_act_RR,offset_Lateral
  Divide{,1,3,5..6} (5 alike) : Product  Inputs=*/
  Gain : Gain  Gain=2
  Product : Product  Inputs=4
  Product1 : Product  Inputs=4
  Product2 : Product  Inputs=4
  Product3 : Product  Inputs=5
  Product4 : Product  Inputs=5
  Product5 : Product  Inputs=6
  Product6 : Product  Inputs=6
  Sum : Sum  Inputs=+-+-
  Sum1 : Sum  Inputs=+---
  Sum2 : Sum  Inputs=++++
  Sum3 : Sum  Inputs=++-+
  Terminator{2..14,16} (14 alike) : Terminator
  const{,1..4} (5 alike) : Constant
  g : Constant  Value=9.81
  h : Constant  Value=0.35
  "l " : Constant  Value=2.745
  l 1 : Constant  Value=2.745*1.684
  l 2 : Constant  Value=2.745*1.7*9.81
  l 3 : Constant  Value=2.745*1.7
  l 4 : Constant  Value=2.745*1.684*9.81
  "lf " : Constant  Value=1.4
  lr : Constant  Value=2.745-1.4
  mass : Constant  Value=1300
  Fz1 : Outport
  Fz2 : Outport  Port=2
  Fz3 : Outport  Port=3
  Fz4 : Outport  Port=4
  wires:
  Product/1 -> Sum1/1, Sum/1  "mglr/2l"
  Product3/1 -> Sum3/3, Sum2/3  "(mayhlf)/(ler)"
  Product2/1 -> Sum2/2, Sum1/2, Sum3/2, Sum/2  "maxh/2l"
  Divide/1 -> Product1/4, Product2/4, Product/4
  Gain/1 -> Divide/2
  const/1 -> Divide/1
  "l "/1 -> Gain/1
  Product1/1 -> Sum3/1, Sum2/1  "mglf/2l"
  "lf "/1 -> Product3/5, Product1/3
  lr/1 -> Product4/4, Product/3
  g/1 -> Product1/1, Product/1
  Bus Selector/7 -> Terminator16/1  "<angRate_Yaw>"
  Bus Selector/4 -> Product6/1, Product5/1, Product4/3, Product3/2  "<acc_Lat>"
  Bus Selector/1 -> Terminator14/1  "<vel_Long>"
  In1/1 -> Bus Selector/1  "feedback"
  Bus Selector/13 -> Terminator9/1  "<wheelTorque_act_FR>"
  Bus Selector/5 -> Terminator2/1  "<angRate_Roll>"
  Bus Selector/14 -> Terminator10/1  "<wheelTorque_act_RL>"
  Bus Selector/11 -> Terminator7/1  "<wheelSpeed_RR>"
  Bus Selector/12 -> Terminator8/1  "<wheelTorque_act_FL>"
  Bus Selector/16 -> Terminator12/1  "<offset_Lateral>"
  Bus Selector/15 -> Terminator11/1  "<wheelTorque_act_RR>"
  Bus Selector/9 -> Terminator5/1  "<wheelSpeed_FR>"
  Bus Selector/8 -> Terminator4/1  "<wheelSpeed_FL>"
  Bus Selector/10 -> Terminator6/1  "<wheelSpeed_RL>"
  Bus Selector/6 -> Terminator3/1  "<angRate_Pitch>"
  Bus Selector/3 -> Product5/3, Product6/3, Product2/2  "<acc_Long>"
  Bus Selector/2 -> Terminator13/1  "<vel_Lat>"
  l 1/1 -> Divide3/2
  const1/1 -> Divide3/1
  Product4/1 -> Sum1/3, Sum/3
  h/1 -> Product2/3, Product6/4, Product6/2, Product5/4, Product5/2, Product4/2, Product3/3
  mass/1 -> Product1/2, Product/2, Product2/1, Product6/5, Product5/5, Product4/1, Product3/1
  const2/1 -> Divide5/1
  l 3/1 -> Divide5/2
  Divide5/1 -> Product4/5
  Divide3/1 -> Product3/4
  const3/1 -> Divide6/1
  l 2/1 -> Divide6/2
  Divide6/1 -> Product5/6
  Product5/1 -> Sum1/4, Sum/4
  Product6/1 -> Sum3/4, Sum2/4
  const4/1 -> Divide1/1
  l 4/1 -> Divide1/2
  Divide1/1 -> Product6/6
  Sum/1 -> Fz1/1
  Sum1/1 -> Fz2/1
  Sum2/1 -> Fz3/1
  Sum3/1 -> Fz4/1

== matlab function solution/Control Algorithm/steer angle block /MATLAB Function ==
  data: xin input; yaw output; yin input; yawdeg output; ex output; ey output
function [yaw,yawdeg,ex,ey]  = yaw_calc(xin,yin)
%syms y  x x0 x1 y0 y1 r

%syms x y r
step=1
%% curve functions
%c1=50+sqrt(r^2-(y-50)^2)-x ;
%c2=50-sqrt(r^2-(y-135)^2)-x;


  ex=0
  ey=0
%% first part of track
if ((yin>-6)&(yin<6))&((xin>=0)&(xin<=50)) %%zalet
    yaw=0;    

elseif ((yin>-6)&(yin<120))&((xin>50)&(xin<200)) %%prvi zavoj
    %p1=((yin-50)/(xin-50))*(x-50)+50-y
    %c11=subs(c1,r,50)
    
    %[xc,yc]=solve([p1;c11])
    xc=[50-50*(1/(xin^2-100*xin+yin^2-100*yin+5000))^(1/2)*(xin-50) ; 50*(1/(xin^2-100*xin+yin^2-100*yin+5000))^(1/2)*(xin-50)+50] 
    yc=[50-50*(1/(xin^2-100*xin+yin^2-100*yin+5000))^(1/2)*(yin-50) ; 50*(1/(xin^2-100*xin+yin^2-100*yin+5000))^(1/2)*(yin-50)+50]
    ynew=yc+step
    
    %xnew=subs(c1+x,[y r],[ynew 50])
    %xnew=subs(c1+x,[y r],[ynew 50])
    xnew=[(2500-(ynew(1)-50)^2)^(1/2)+50 ; (2500-(ynew(2)-50)^2)^(1/2)+50]
    
    %vpa([xc yc])
    %vpa([xnew ynew])
    
    %rjjjjj=(solve(c1,y))
    
    %cldiff=diff(solve(c1,y))
    cldiff1=[-(2*xnew(1)-100)/(2*(-xnew(1)*(xnew(1)-100))^(1/2)) ; (2*xnew(1)-100)/(2*(-xnew(1)*(xnew(1)-100))^(1/2))]
    %cldiff2=[-(2*xnew(2)-100)/(2*(-xnew(2)*(xnew(2)-100))^(1/2)) ; (2*xnew(2)-100)/(2*(-xnew(2)*(xnew(2)-100))^(1/2))]
    cldiff=[cldiff1(2)]%; cldiff2]
    if (not(xnew==50+50))
    %tanyaw=subs(cldiff(2),[r x],[50 xnew])
    tanyaw=cldiff
    else
        tanyaw=inf
    end
    yaw=atand(tanyaw)
    if((xnew(2)<=100)&(ynew(2)>50))
        yaw=180-yaw
    end
    %vpa(yaw)
    %yaw=11;

    %ex=0
    %ey=0
    
elseif ((yin>94)&(yin<176))&((xin<=50)&(xin>9)) %%drugi zavoj
   %p2=((yin-135)/(xin-50))*(x-50)+135-y
   %c22=subs(c2,r,35)
    
    %[xc,yc]=solve([p2;c22])
    xc=[50-35*(1/(xin^2-100*xin+yin^2-270*yin+20725))^(1/2)*(xin-50) ;   35*(1/(xin^2-100*xin+yin^2-270*yin+20725))^(1/2)*(xin-50)+50]
    yc=[135-35*(1/(xin^2-100*xin+yin^2-270*yin+20725))^(1/2)*(yin-135) ; 35*(1/(xin^2-100*xin+yin^2-270*yin+20725))^(1/2)*(yin-135)+135]
    ynew=yc+step
    
    
    %xnew=subs(c2+x,[y r],[ynew 35])
    xnew=[50-(1225-(ynew(1)-135)^2)^(1/2) ; 50-(1225-(ynew(2)-135)^2)^(1/2)]
   
    %vpa([xc yc])
    %vpa([xnew ynew])
    
    %cldiff=diff(solve(c2,y))
    cldiff1=[-(2*xnew(1)-100)/(2*(-(xnew(1)-15)*(xnew(1)-85))^(1/2)) ; (2*xnew(1)-100)/(2*(-(xnew(1)-15)*(xnew(1)-85))^(1/2))]
    cldiff2=[-(2*xnew(2)-100)/(2*(-(xnew(2)-15)*(xnew(2)-85))^(1/2)) ; (2*xnew(2)-100)/(2*(-(xnew(2)-15)*(xnew(2)-85))^(1/2))]
    
    cldiff=[cldiff1(1)]
    
    if (not(xnew==50-35))
    tanyaw=cldiff
    else
        tanyaw=inf
    end
    yaw=atand(tanyaw)
    if((xnew(2)>15)&(ynew(2)>135))
        yaw=yaw
        disp('sl 2')
    else
        yaw=180-yaw
        disp('sl 1')
    end
    
    %kut=vpa(yaw)
    disp('drugi')
    %yaw=-11
    
    %ex=0
    %ey=0
elseif ((yin>94)&(yin<176))&((xin>50)&(xin<=100)) %zaustavljanje
    yaw=0
    ex=xin
    ey=yin
else
    yaw=55
    ex=xin
    ey=yin

end
yawdeg=yaw
yaw=yaw*pi/180


end
